simulink model "mysim2"  (R2018b)
settings: Solver=FixedStepDiscrete  StartTime=0.0  StopTime=6.28  FixedStep=0.001  RelTol=1e-3
settings Model: Creator=Billy  LastModifiedBy=Billy
settings DataIOCC: SaveFormat=Array

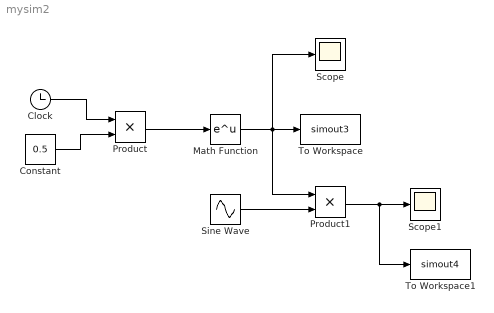
== system mysim2 ==
  Clock : Clock
  Constant : Constant  Value=0.5
  Math Function : Math  SaturateOnIntegerOverflow=on
  Product : Product
  Product1 : Product
  Scope : Scope
  Scope1 : Scope
  Sine Wave : Sin  Frequency=2  SampleTime=0
  To Workspace : ToWorkspace  VariableName=simout3  SaveFormat=Timeseries  SampleTime=-1
  To Workspace1 : ToWorkspace  VariableName=simout4  SaveFormat=Timeseries  SampleTime=-1
  wires:
  Clock/1 -> Product/1
  Constant/1 -> Product/2
  Product/1 -> Math Function/1
  Math Function/1 -> Product1/1, Scope/1, To Workspace/1
  Sine Wave/1 -> Product1/2
  Product1/1 -> To Workspace1/1, Scope1/1
